simulink model "Week3_Problem3"  (R2020b)
settings: Solver=VariableStepAuto  StartTime=0.0  StopTime=25  RelTol=1e-3
model workspace (MAT data in the model file):
  I = Simulink.Parameter
  I.Value = 5
  I.DataType = 'auto'
  I.Dimensions = [1 1]
  R = Simulink.Parameter
  R.Value = 1.25
  R.DataType = 'auto'
  R.Dimensions = [1 1]
  g = Simulink.Parameter
  g.Value = 9.81
  g.DataType = 'auto'
  g.Dimensions = [1 1]
  m = Simulink.Parameter
  m.Value = 5
  m.DataType = 'auto'
  m.Dimensions = [1 1]
  v0 = Simulink.Parameter
  v0.Value = 88
  v0.DataType = 'auto'
  v0.Dimensions = [1 1]
settings Model: Creator=ASUS  LastModifiedBy=ASUS

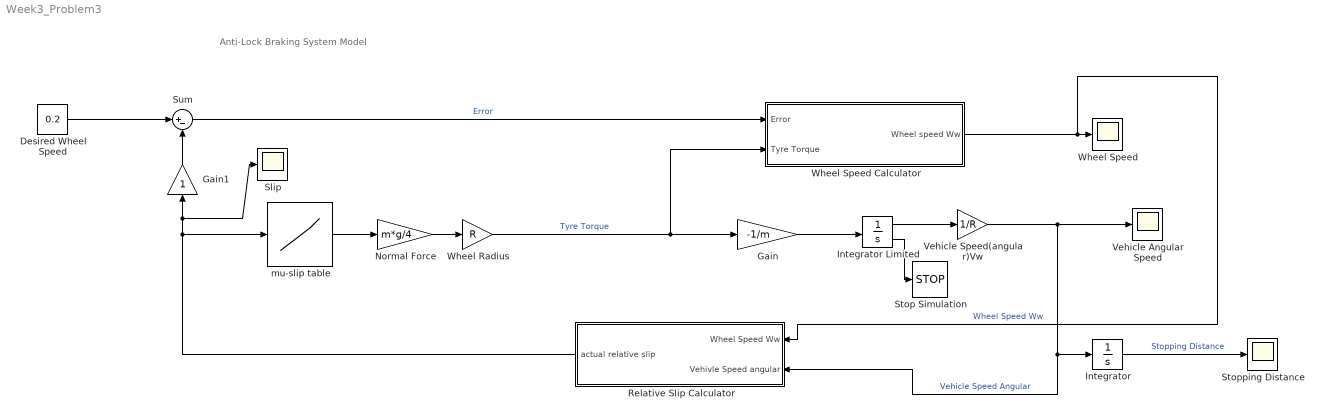
== system Week3_Problem3 ==
  note: Anti-Lock Braking System Model
  Desired Wheel Speed : Constant  Value=0.2
  Gain : Gain  Gain=-1/m
  Gain1 : Gain
  Integrator : Integrator
  Integrator Limited : Integrator  InitialCondition=v0  LimitOutput=on  UpperSaturationLimit=1000  LowerSaturationLimit=0  ShowSaturationPort=on
  Normal Force : Gain  Gain=m*g/4
  Relative Slip Calculator : Subsystem
  Slip : Scope
  Stop Simulation : Stop
  Stopping Distance : Scope
  Sum : Sum  Inputs=|+-
  Vehicle Angular Speed : Scope
  Vehicle Speed(angular)Vw : Gain  Gain=1/R
  Wheel Radius : Gain  Gain=R
  Wheel Speed : Scope
  Wheel Speed Calculator : Subsystem
  mu-slip table : Lookup_n-D  NumberOfTableDimensions=1  BreakpointsForDimension1=[0,0.05,0.1,0.15,0.2,0.25,0.3,0.35,0.4,0.45,.5,0.55,0.6,0.65,0.7,0.75,0.8,0.85,0.9,0.95,1]  Table=[0,0.4,0.8,0.97,1,0.98,0.96,0.94,0.92,0.9,0.88,0.855,0.83,0.81,0.79,0.77,0.75,0.73,0.72,0.71,0.7]  InternalRulePriority=Speed  RndMeth=Simplest  InputSameDT=on
  wires:
  Desired Wheel Speed/1 -> Sum/1
  mu-slip table/1 -> Normal Force/1
  Normal Force/1 -> Wheel Radius/1
  Sum/1 -> Wheel Speed Calculator/1(Error)  "Error"
  Wheel Radius/1 -> Gain/1, Wheel Speed Calculator/2(Tyre Torque)  "Tyre Torque"
  Wheel Speed Calculator/1(Wheel speed Ww) -> Wheel Speed/1, Relative Slip Calculator/1(Wheel Speed Ww)  "Wheel Speed Ww"
  Gain/1 -> Integrator Limited/1
  Integrator Limited/1 -> Vehicle Speed(angular)Vw/1
  Vehicle Speed(angular)Vw/1 -> Integrator/1, Relative Slip Calculator/2(Vehivle Speed angular), Vehicle Angular Speed/1  "Vehicle Speed Angular"
  Integrator Limited/2 -> Stop Simulation/1
  Relative Slip Calculator/1(actual relative slip) -> Gain1/1, Slip/1, mu-slip table/1
  Integrator/1 -> Stopping Distance/1  "Stopping Distance"
  Gain1/1 -> Sum/2

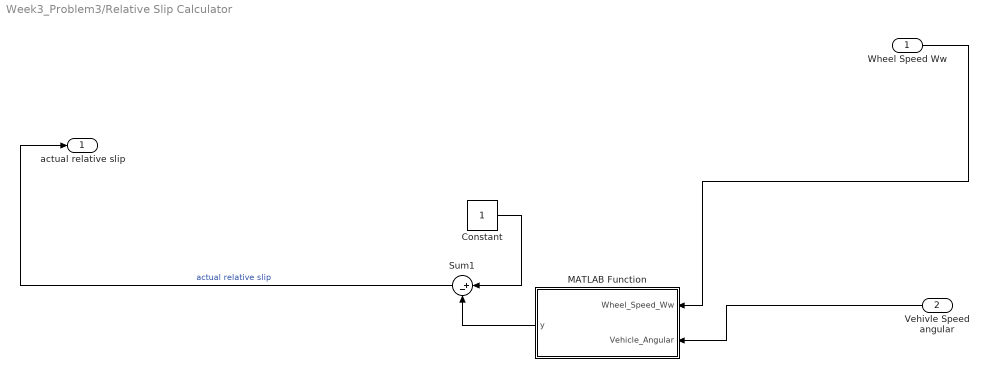
== system Week3_Problem3/Relative Slip Calculator ==
  Wheel Speed Ww : Inport
  Vehivle Speed angular : Inport  Port=2
  Constant : Constant
  MATLAB Function : MATLAB Function  TreatAsAtomicUnit=on
  Sum1 : Sum  Inputs=|+-
  actual relative slip : Outport
  wires:
  MATLAB Function/1(y) -> Sum1/2
  Wheel Speed Ww/1 -> MATLAB Function/1(Wheel_Speed_Ww)
  Sum1/1 -> actual relative slip/1  "actual relative slip"
  Constant/1 -> Sum1/1
  Vehivle Speed angular/1 -> MATLAB Function/2(Vehicle_Angular)

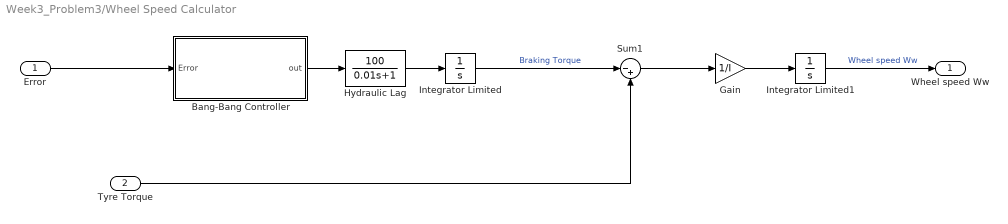
== system Week3_Problem3/Wheel Speed Calculator ==
  Error : Inport
  Tyre Torque : Inport  Port=2
  Bang-Bang Controller : Subsystem
  Gain : Gain  Gain=1/I
  Hydraulic Lag : TransferFcn  Numerator=[100]  Denominator=[0.01 1]
  Integrator Limited : Integrator  LimitOutput=on  UpperSaturationLimit=1000  LowerSaturationLimit=0
  Integrator Limited1 : Integrator  InitialCondition=v0/R  LimitOutput=on  UpperSaturationLimit=1000  LowerSaturationLimit=0
  Sum1 : Sum  Inputs=|-+
  Wheel speed Ww : Outport
  wires:
  Hydraulic Lag/1 -> Integrator Limited/1
  Gain/1 -> Integrator Limited1/1
  Error/1 -> Bang-Bang Controller/1(Error)
  Bang-Bang Controller/1(out) -> Hydraulic Lag/1
  Integrator Limited1/1 -> Wheel speed Ww/1  "Wheel speed Ww"
  Integrator Limited/1 -> Sum1/1  "Braking Torque"
  Tyre Torque/1 -> Sum1/2
  Sum1/1 -> Gain/1

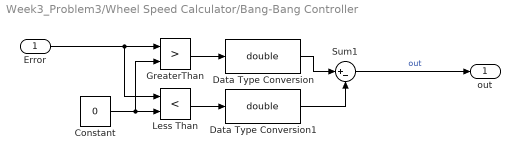
== system Week3_Problem3/Wheel Speed Calculator/Bang-Bang Controller ==
  Error : Inport
  Constant : Constant  Value=0
  Data Type Conversion : DataTypeConversion  OutDataTypeStr=double  RndMeth=Zero
  Data Type Conversion1 : DataTypeConversion  OutDataTypeStr=double  RndMeth=Zero
  GreaterThan : RelationalOperator  Operator=>  OutDataTypeStr=boolean  RndMeth=Simplest
  Less Than : RelationalOperator  Operator=<  OutDataTypeStr=boolean  RndMeth=Simplest
  Sum1 : Sum  Inputs=|+-
  out : Outport
  wires:
  Error/1 -> Less Than/1, GreaterThan/1
  Data Type Conversion/1 -> Sum1/1
  Less Than/1 -> Data Type Conversion1/1
  Constant/1 -> GreaterThan/2, Less Than/2
  GreaterThan/1 -> Data Type Conversion/1
  Data Type Conversion1/1 -> Sum1/2
  Sum1/1 -> out/1  "out"

== matlab function Week3_Problem3/Relative Slip Calculator/MATLAB Function ==
  data: Wheel_Speed_Ww input; Vehicle_Angular input; y output
function y = fcn(Wheel_Speed_Ww, Vehicle_Angular)

y = Wheel_Speed_Ww/Vehicle_Angular
